simulink model "ForwardKinematic_YuMi"  (R2024a)
(part 23 of 23)

(7514214926474921*cos(q2R)*((3148506117433717*cos(q1R))/4503599627370496 + (1211728953682539*sin(q1R))/2251799813685248))/36893488147419103232 - sin(q2R)*((1211728953682539*cos(q1R))/2251799813685248 - (3148506117433717*sin(q1R))/4503599627370496)))/36893488147419103232 + sin(q3R)*((4774755754024928798560446539205*sin(q2R))/10141204801825835211973625643008 + cos(q2R)*((1211728953682539*cos(q1R))/2251799813685248 - (3148506117433717*sin(q1R))/4503599627370496) + (7514214926474921*sin(q2R)*((3148506117433717*cos(q1R))/4503599627370496 + (1211728953682539*sin(q1R))/2251799813685248))/36893488147419103232) + (9007199067919185*cos(q3R)*((28359221366286827792295350160645*cos(q1R))/40564819207303340847894502572032 + (10914283902180054573281797610715*sin(q1R))/20282409603651670423947251286016 - 3983318308679801924058395430653/41538374868278621028243970633760768))/9007199254740992))/36893488147419103232) + (9007199067919185*cos(q5R)*((67399765602155231606998903473897443684277400996768941497011875*cos(q2R))/3450873173395281893717377931138512726225554486085193277581262111899648 - (333960713126929533372903469589741180908441336378844163830032875*cos(q1R))/56539106072908298546665520023773392506479484700019806659891398441363832832 - (128527577967104929471702655059245076724477257328642562920515125*sin(q1R))/28269553036454149273332760011886696253239742350009903329945699220681916416 + (106069577339469832923929692356850887620017617375*cos(q2R)*((3148506117433717*cos(q1R))/4503599627370496 + (1211728953682539*sin(q1R))/2251799813685248))/12554203470773361527671578846415332832204710888928069025792 + (67682029681889335677290557259385*cos(q3R)*((4774755754024928798560446539205*cos(q2R))/10141204801825835211973625643008 + (7514214926474921*cos(q2R)*((3148506117433717*cos(q1R))/4503599627370496 + (1211728953682539*sin(q1R))/2251799813685248))/36893488147419103232 - sin(q2R)*((1211728953682539*cos(q1R))/2251799813685248 - (3148506117433717*sin(q1R))/4503599627370496)))/332306998946228968225951765070086144 - (14115856197532180673579726082375*sin(q2R)*((1211728953682539*cos(q1R))/2251799813685248 - (3148506117433717*sin(q1R))/4503599627370496))/340282366920938463463374607431768211456 + (234819211581865*cos(q3R)*((4774755754024928798560446539205*sin(q2R))/10141204801825835211973625643008 + cos(q2R)*((1211728953682539*cos(q1R))/2251799813685248 - (3148506117433717*sin(q1R))/4503599627370496) + (7514214926474921*sin(q2R)*((3148506117433717*cos(q1R))/4503599627370496 + (1211728953682539*sin(q1R))/2251799813685248))/36893488147419103232))/1152921504606846976 - (1764482024691522628700660907665*sin(q3R)*((4774755754024928798560446539205*cos(q2R))/10141204801825835211973625643008 + (7514214926474921*cos(q2R)*((3148506117433717*cos(q1R))/4503599627370496 + (1211728953682539*sin(q1R))/2251799813685248))/36893488147419103232 - sin(q2R)*((1211728953682539*cos(q1R))/2251799813685248 - (3148506117433717*sin(q1R))/4503599627370496)))/42535295865117307932921825928971026432 + (9007199067919185*sin(q3R)*((4774755754024928798560446539205*sin(q2R))/10141204801825835211973625643008 + cos(q2R)*((1211728953682539*cos(q1R))/2251799813685248 - (3148506117433717*sin(q1R))/4503599627370496) + (7514214926474921*sin(q2R)*((3148506117433717*cos(q1R))/4503599627370496 + (1211728953682539*sin(q1R))/2251799813685248))/36893488147419103232))/9007199254740992 + (81129635049124235038645691064225*cos(q3R)*((28359221366286827792295350160645*cos(q1R))/40564819207303340847894502572032 + (10914283902180054573281797610715*sin(q1R))/20282409603651670423947251286016 - 3983318308679801924058395430653/41538374868278621028243970633760768))/81129638414606681695789005144064 - (2115063383689692319117831580025*sin(q3R)*((28359221366286827792295350160645*cos(q1R))/40564819207303340847894502572032 + (10914283902180054573281797610715*sin(q1R))/20282409603651670423947251286016 - 3983318308679801924058395430653/41538374868278621028243970633760768))/10384593717069655257060992658440192 + 46907910686140203564236702804319721336174201386222453025052275/57896044618658097711785492504343953926634992332820282019728792003956564819968))/9007199254740992 + (7514214926474921*cos(q5R)*(((4503599440548691*cos(q4R))/4503599627370496 - (7514214926474921*sin(q4R))/36893488147419103232)*((7514214926474921*sin(q3R)*((4774755754024928798560446539205*cos(q2R))/10141204801825835211973625643008 + (7514214926474921*cos(q2R)*((3148506117433717*cos(q1R))/4503599627370496 + (1211728953682539*sin(q1R))/2251799813685248))/36893488147419103232 - sin(q2R)*((1211728953682539*cos(q1R))/2251799813685248 - (3148506117433717*sin(q1R))/4503599627370496)))/36893488147419103232 - cos(q3R)*((4774755754024928798560446539205*sin(q2R))/10141204801825835211973625643008 + cos(q2R)*((1211728953682539*cos(q1R))/2251799813685248 - (3148506117433717*sin(q1R))/4503599627370496) + (7514214926474921*sin(q2R)*((3148506117433717*cos(q1R))/4503599627370496 + (1211728953682539*sin(q1R))/2251799813685248))/36893488147419103232) + (9007199067919185*sin(q3R)*((28359221366286827792295350160645*cos(q1R))/40564819207303340847894502572032 + (10914283902180054573281797610715*sin(q1R))/20282409603651670423947251286016 - 3983318308679801924058395430653/41538374868278621028243970633760768))/9007199254740992) + ((234819211581865*cos(q4R))/1152921504606846976 + (9007199067919185*sin(q4R))/9007199254740992)*((213097284493758984364555654519459856780913684045*cos(q1R))/1496577676626844588240573268701473812127674924007424 - (43007175577195104036898489188735438973874147925*cos(q2R))/91343852333181432387730302044767688728495783936 + (82012275009546312639155898108543355135168378515*sin(q1R))/748288838313422294120286634350736906063837462003712 - (67682029681889335677290557259385*cos(q2R)*((3148506117433717*cos(q1R))/4503599627370496 + (1211728953682539*sin(q1R))/2251799813685248))/332306998946228968225951765070086144 + (9007199067919185*sin(q2R)*((1211728953682539*cos(q1R))/2251799813685248 - (3148506117433717*sin(q1R))/4503599627370496))/9007199254740992 - 29931509891982604486959633650198707742999153413/1532495540865888858358347027150309183618739122183602176) + (7514214926474921*cos(q4R)*((7514214926474921*cos(q3R)*((4774755754024928798560446539205*cos(q2R))/10141204801825835211973625643008 + (7514214926474921*cos(q2R)*((3148506117433717*cos(q1R))/4503599627370496 + (1211728953682539*sin(q1R))/2251799813685248))/36893488147419103232 - sin(q2R)*((1211728953682539*cos(q1R))/2251799813685248 - (3148506117433717*sin(q1R))/4503599627370496)))/36893488147419103232 + sin(q3R)*((4774755754024928798560446539205*sin(q2R))/10141204801825835211973625643008 + cos(q2R)*((1211728953682539*cos(q1R))/2251799813685248 - (3148506117433717*sin(q1R))/4503599627370496) + (7514214926474921*sin(q2R)*((3148506117433717*cos(q1R))/4503599627370496 + (1211728953682539*sin(q1R))/2251799813685248))/36893488147419103232) + (9007199067919185*cos(q3R)*((28359221366286827792295350160645*cos(q1R))/40564819207303340847894502572032 + (10914283902180054573281797610715*sin(q1R))/20282409603651670423947251286016 - 3983318308679801924058395430653/41538374868278621028243970633760768))/9007199254740992))/36893488147419103232))/36893488147419103232))/36893488147419103232000, 0];
end
